simulink model "aero_six_dof"  (Simulink 6.0)
settings: Solver=ode45  SolverMode=SingleTasking  StartTime=0.0  StopTime=10  MaxStep=0.02  RelTol=1e-5  AbsTol=1e-7
libraries: simulink x6, aerospace x1
settings Model: CovMetricSettings=d  Creator=The MathWorks Inc.  LastModifiedBy=batserve  ExtModeTrigMode=oneshot  ExtModeArmWhenConnect=off  ExtModeAutoUpdateStatusClock=off
settings DataIOCC: LimitDataPoints=off  SaveOutput=off  SignalLoggingName=sigsOut
settings OptimizationCC: BlockReduction=off  BooleanDataType=off
settings DebuggingCC: CheckExecutionContextPreStartOutputMsg=on  CheckExecutionContextRuntimeOutputMsg=on  SolverPrmCheckMsg=none
settings HardwareCC: TargetUnknown=on
settings RTWCC: TemplateMakefile=grt_vc.tmf

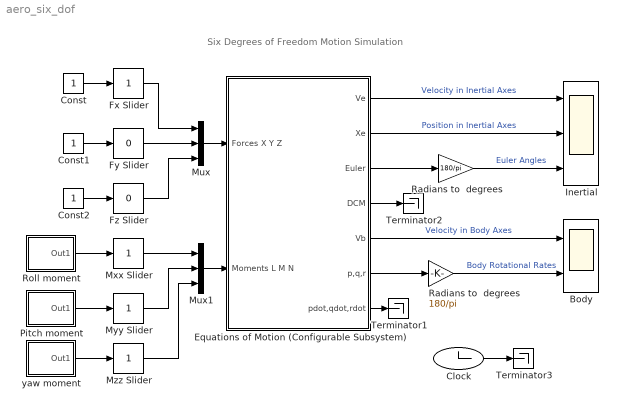
== system aero_six_dof ==
  note: Six Degrees of Freedom Motion Simulation
  Body : Scope  NumInputPorts=2
      settings: TimeRange=10  YMin=-2~-100  YMax=6~100
  Clock : Clock
      settings: Decimation=100
  Const : Constant
  Const1 : Constant
  Const2 : Constant
  Equations of Motion (Configurable Subsystem) : Subsystem  BlockChoice=Euler Angles  PropExecContextAcrossSSBoundary=on
      settings: MemberBlocks=Euler Angles,Quaternions
      settings: TemplateBlock=|
      | aerospace/6DoF/Equations of Motion
      | (Configurable Subsystem)
  Fx Slider : simulink/Math Operations/Slider Gain  low=-1  gain=1  high=1
  Fy Slider : simulink/Math Operations/Slider Gain  low=-1  gain=0  high=1
  Fz Slider : simulink/Math Operations/Slider Gain  low=-1  gain=0  high=1
  Inertial : Scope  NumInputPorts=3
      settings: TickLabels=on  TimeRange=10  YMin=-2~-10~-50  YMax=6~40~100  SaveName=InertialData
  Mux : Mux  Inputs=3
  Mux1 : Mux  Inputs=3
  Mxx Slider : simulink/Math Operations/Slider Gain  low=-5  gain=1  high=10
  Myy Slider : simulink/Math Operations/Slider Gain  low=-10  gain=1  high=10
  Mzz Slider : simulink/Math Operations/Slider Gain  low=-1  gain=1  high=1
  Pitch moment : Subsystem  PropExecContextAcrossSSBoundary=on  mask(timed input){t=[0 3 3 4 4 5 5  7.5 7.5 8.5 8.5 9.5 9.5 10], u=[0 0  1 1 -1 -1.005 0 0 -1 -1 1 1 0 0]*3.138/2}
      mask prompts: t "time values:"; u "input values"
      mask Display: plot(t,u)
  Radians to  degrees : Gain  Gain=180/pi  SaturateOnIntegerOverflow=on
  "Radians to  degrees " : Gain  Gain=180/pi  SaturateOnIntegerOverflow=on
  Roll moment : Subsystem  PropExecContextAcrossSSBoundary=on  mask(timed input){t=[0 1 1 2 2  10], u=[1 1 -1 -.998  0 0]*3.144/2}
      mask prompts: t "time values:"; u "input values"
      mask Display: plot(t,u)
  Terminator1 : Terminator
  Terminator2 : Terminator
  Terminator3 : Terminator
  yaw moment : Subsystem  PropExecContextAcrossSSBoundary=on  mask(timed input){t=[0 6 6 7 7 8 8 10], u=[0 0  -1 -1 1 1 0 0]*3.1/2}
      mask prompts: t "time values:"; u "input values"
      mask Display: plot(t,u)
  wires:
  yaw moment/1(Out1) -> Mzz Slider/1
  Pitch moment/1(Out1) -> Myy Slider/1
  Roll moment/1(Out1) -> Mxx Slider/1
  Const2/1 -> Fz Slider/1
  Const1/1 -> Fy Slider/1
  Const/1 -> Fx Slider/1
  Clock/1 -> Terminator3/1
  Mux1/1 -> Equations of Motion (Configurable Subsystem)/2(Moments L M N)
  Mzz Slider/1 -> Mux1/3
  Myy Slider/1 -> Mux1/2
  Mxx Slider/1 -> Mux1/1
  Mux/1 -> Equations of Motion (Configurable Subsystem)/1(Forces X Y Z)
  Fy Slider/1 -> Mux/2
  Fz Slider/1 -> Mux/3
  Fx Slider/1 -> Mux/1
  Equations of Motion (Configurable Subsystem)/4(DCM) -> Terminator2/1
  Equations of Motion (Configurable Subsystem)/7(pdot,qdot,rdot) -> Terminator1/1
  Equations of Motion (Configurable Subsystem)/3(Euler) -> Radians to  degrees/1
  Equations of Motion (Configurable Subsystem)/5(Vb) -> Body/1  "Velocity in Body Axes"
  Equations of Motion (Configurable Subsystem)/1(Ve) -> Inertial/1  "Velocity in Inertial Axes"
  Equations of Motion (Configurable Subsystem)/2(Xe) -> Inertial/2  "Position in Inertial Axes"
  Radians to  degrees/1 -> Inertial/3  "Euler Angles"
  Equations of Motion (Configurable Subsystem)/6(p,q,r) -> "Radians to  degrees "/1
  "Radians to  degrees "/1 -> Body/2  "Body Rotational Rates"

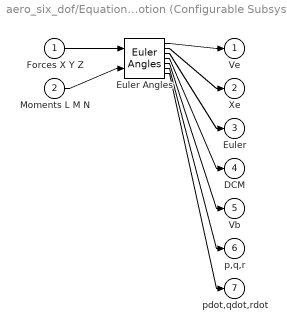
== system aero_six_dof/Equations of Motion (Configurable Subsystem) ==
  Forces X Y Z : Inport  Port=1  LatchInput=off
  Moments L M N : Inport  Port=2  LatchInput=off
  Euler Angles : aerospace/6DoF/Euler Angles  xme_0=[0 0 0]  Vm_0=[0 0 0]  eul_0=[0 0 0]  pm_0=[0 0 0]  Mass=1.0  Inertia=eye(3)
  Ve : Outport
  Xe : Outport  Port=2
  Euler : Outport  Port=3
  DCM : Outport  Port=4
  Vb : Outport  Port=5
  p,q,r : Outport  Port=6
  pdot,qdot,rdot : Outport  Port=7
  wires:
  Forces X Y Z/1 -> Euler Angles/1
  Moments L M N/1 -> Euler Angles/2
  Euler Angles/1 -> Ve/1
  Euler Angles/2 -> Xe/1
  Euler Angles/3 -> Euler/1
  Euler Angles/4 -> DCM/1
  Euler Angles/5 -> Vb/1
  Euler Angles/6 -> p,q,r/1
  Euler Angles/7 -> pdot,qdot,rdot/1

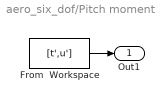
== system aero_six_dof/Pitch moment ==
  From  Workspace : FromWorkspace  VariableName=[t',u']  SampleTime=0
  Out1 : Outport  InitialOutput=0
  wires:
  From  Workspace/1 -> Out1/1

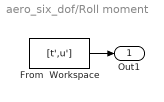
== system aero_six_dof/Roll moment ==
  From  Workspace : FromWorkspace  VariableName=[t',u']  SampleTime=0
  Out1 : Outport  InitialOutput=0
  wires:
  From  Workspace/1 -> Out1/1

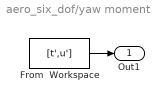
== system aero_six_dof/yaw moment ==
  From  Workspace : FromWorkspace  VariableName=[t',u']  SampleTime=0
  Out1 : Outport  InitialOutput=0
  wires:
  From  Workspace/1 -> Out1/1
